simulink model "linearpendulum"  (R2018b)
settings: Solver=VariableStepAuto  StartTime=0.0  StopTime=5  RelTol=1e-3
values from neighbouring files (symbols this model uses):
  A = [0 1 0 0 ... (first row only)    [Pendulum.m]    (also in init_cranedamping.m = [0 1 0 0; 0 0 0 0; 0 0 0 1; 0 0 -g/l 1]; init_cranedamping_lqr.m)
  B = [0 1 0 1/l]'    [Pendulum.m]    (also in init_cranedamping.m = [0; 1; 0; 1/l]; init_cranedamping_lqr.m)
  C = eye(4)    [Pendulum.m]    (also in init_cranedamping.m = [ 1 0 0 0; 0 0 1 0]; init_cranedamping_lqr.m = [ 1 0 0 0; 0 0 0 0; 0 0 1 0; 0 0 0 0])
  ctrl = lqr(A,B,Q,R)    [Pendulum.m]    (also in init_cranedamping_lqr.m)
  ref = 0    [Pendulum.m]    (also in init_cranedamping_lqr.m)
  theta_0 = pi/2    (= 1.57079632679)    [Pendulum.m]    (also in init_cranedamping_lqr.m)
settings Model: Creator=ola  LastModifiedBy=ola

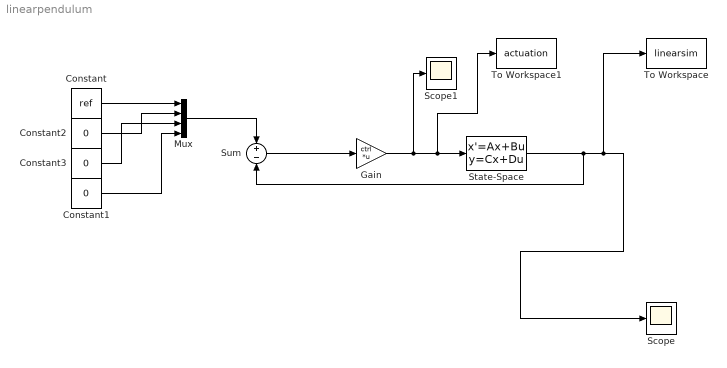
== system linearpendulum ==
  Constant : Constant  Value=ref
  Constant1 : Constant  Value=0
  Constant2 : Constant  Value=0
  Constant3 : Constant  Value=0
  Gain : Gain  Gain=ctrl  Multiplication=Matrix(K*u) (u vector)
  Mux : Mux
  Scope : Scope
  Scope1 : Scope
  State-Space : StateSpace  A=A  B=B  C=C  D=[0 0 0 0]'  InitialCondition=[0 0 theta_0 0]
  Sum : Sum  Inputs=+-
  To Workspace : ToWorkspace  VariableName=linearsim  SaveFormat=Timeseries  SampleTime=-1
  To Workspace1 : ToWorkspace  VariableName=actuation  SaveFormat=Timeseries  SampleTime=-1
  wires:
  State-Space/1 -> Sum/2, To Workspace/1, Scope/1
  Gain/1 -> Scope1/1, To Workspace1/1, State-Space/1
  Sum/1 -> Gain/1
  Mux/1 -> Sum/1
  Constant/1 -> Mux/1
  Constant2/1 -> Mux/2
  Constant3/1 -> Mux/3
  Constant1/1 -> Mux/4
